simulink model "unwrapper"  (Simulink 3.00)
settings: Solver=ode45  StartTime=0.0  StopTime=10.0  RelTol=1e-3
libraries: simulink3 x1
settings Model: BooleanDataType=on  ExtModeTrigMode=normal  ExtModeArmWhenConnect=on  LastModifiedBy=campa

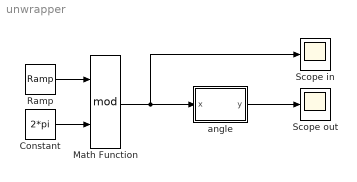
== system unwrapper ==
  Constant : Constant  Value=2*pi
  Math Function : Math  Operator=mod  OutputSignalType=auto
  Ramp : simulink3/Sources/Ramp  slope=1  start=0  X0=0
  Scope in : Scope
      settings: TimeRange=10  YMin=0  YMax=10  SaveToWorkspace=off
  Scope out : Scope
      settings: TimeRange=10  YMin=0  YMax=10  SaveToWorkspace=off  SaveName=ScopeData
  angle : Subsystem  mask(Unwrap Angle){L=4, x0=0, T=0.005}
      mask prompts: L "Maximum angular distance covered during the sample time (< 2*pi)"; x0 "Initial Input"; T "Sample Time"
      mask help:
      | The output angle does not make 2*pi wide jumps.
      |   It is assumed that, with the exception of the jumps,
      |   the maximum magnitude of the time derivative of the input
      |   is less than L/T [rad/sec], where L and T are the first and third
      |   parameters in the mask.
      mask Help:
      | The output angle does not make 2*pi wide jumps.
      |   It is assumed that, with the exception of the jumps,
      |   the maximum magnitude of the time derivative of the input
      |   is less than L/T [rad/sec], where L and T are the first and third
      |   parameters in the mask.
      mask Display: disp('UnWrap')
  wires:
  Ramp/1 -> Math Function/1
  Constant/1 -> Math Function/2
  Math Function/1 -> Scope in/1, angle/1(x)
  angle/1(y) -> Scope out/1

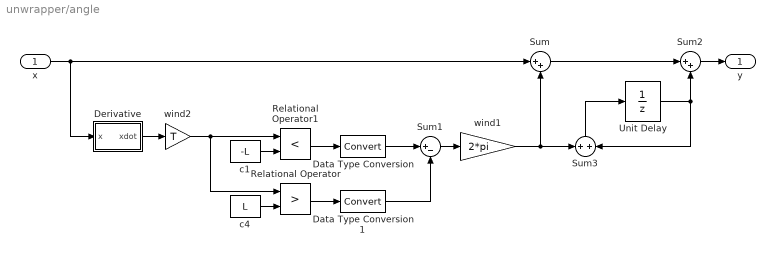
== system unwrapper/angle ==
  x : Inport  Port=1  PortWidth=-1  SampleTime=-1  DataType=auto
      settings: SignalType=auto
  Data Type Conversion : DataTypeConversion  DataType=double  SaturateOnIntegerOverflow=on
  Data Type Conversion1 : DataTypeConversion  DataType=double  SaturateOnIntegerOverflow=on
  Derivative : Subsystem  mask(Time Derivative){T=T, x0=x0}
      mask prompts: T "Sampling Time"; x0 "Initial Condition"
      mask help:
      | First order approximation of the time derivative of the input signal,
      |   the original one is buggy.
  Relational Operator : RelationalOperator  Operator=>
  Relational Operator1 : RelationalOperator  Operator=<
  Sum : Sum  Inputs=|++  SaturateOnIntegerOverflow=on
  Sum1 : Sum  Inputs=|+-  SaturateOnIntegerOverflow=on
  Sum2 : Sum  Inputs=|++  SaturateOnIntegerOverflow=on
  Sum3 : Sum  Orientation=up  Inputs=++  SaturateOnIntegerOverflow=on
  Unit Delay : UnitDelay  X0=0  SampleTime=T
  c1 : Constant  Value=-L
  c4 : Constant  Value=L
  wind1 : Gain  Gain=2*pi  SaturateOnIntegerOverflow=on
  wind2 : Gain  Gain=T  SaturateOnIntegerOverflow=on
  y : Outport  Port=1
  wires:
  Derivative/1(xdot) -> wind2/1
  wind2/1 -> Relational Operator/1, Relational Operator1/1
  c4/1 -> Relational Operator/2
  c1/1 -> Relational Operator1/2
  Relational Operator1/1 -> Data Type Conversion/1
  Relational Operator/1 -> Data Type Conversion1/1
  Data Type Conversion/1 -> Sum1/1
  Data Type Conversion1/1 -> Sum1/2
  Sum1/1 -> wind1/1
  wind1/1 -> Sum/2, Sum3/1
  Sum/1 -> Sum2/1
  Unit Delay/1 -> Sum2/2, Sum3/2
  Sum3/1 -> Unit Delay/1
  Sum2/1 -> y/1
  x/1 -> Sum/1, Derivative/1(x)

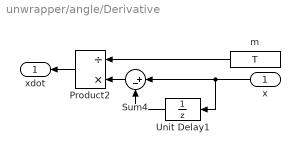
== system unwrapper/angle/Derivative ==
  x : Inport  Orientation=left  Port=1  PortWidth=-1  SampleTime=T  DataType=auto
      settings: SignalType=auto
  Product2 : Product  Orientation=left  Inputs=/*  SaturateOnIntegerOverflow=on
  Sum4 : Sum  Orientation=left  Inputs=|+-  SaturateOnIntegerOverflow=on
  Unit Delay1 : UnitDelay  Orientation=left  X0=x0  SampleTime=T
  m : Constant  Orientation=left  Value=T
  xdot : Outport  Orientation=left  Port=1
  wires:
  Product2/1 -> xdot/1
  m/1 -> Product2/1
  x/1 -> Unit Delay1/1, Sum4/1
  Unit Delay1/1 -> Sum4/2
  Sum4/1 -> Product2/2
